simulink library "halout"  (R2021b)
settings: Solver=VariableStepAuto  StartTime=0.0  StopTime=10.0  RelTol=1e-3
undefined symbols (not defined in the file): C_TASK_5MS_S, FALSE, KHAL_CAN1FD1APS3E2E_flg, KHAL_CAN1FD1APS3TxReq_flg, KHAL_CAN1FD1VCU2E2E_flg, KHAL_CAN1FD1VCU2TxReq_flg, KHAL_CAN1FD1VCU3E2E_flg, KHAL_CAN1FD1VCU3TxReq_flg, KHAL_CAN1TxReq_flg, KHAL_CAN1VMCFCM1E2E_flg, KHAL_CAN1VMCFCM1TxReq_flg, KHAL_CAN2TxReq_flg, KHAL_CAN3FD3VCU1toNIDECTxReq_flg, KHAL_CAN3FD3VCU1TxReq_flg, KHAL_CAN3FD3VCU2E2E_flg, KHAL_CAN3FD3VCU2toNIDECE2E_flg, KHAL_CAN3FD3VCU2toNIDECTxReq_flg, KHAL_CAN3FD3VCU2TxReq_flg, KHAL_CAN3TxReq_flg, KHAL_CAN4FD4CE1000E2E_flg, KHAL_CAN4FD4CE1000TxReq_flg, KHAL_CAN4TxReq_flg, KHAL_CAN5TxReq_flg, KHAL_CAN6FD6APS3E2E_flg, KHAL_CAN6FD6APS3TxReq_flg, KHAL_CAN6FD6VCU2E2E_flg, KHAL_CAN6FD6VCU2TxReq_flg, KHAL_CAN6TxReq_flg, ONE_INT, TRUE, ZERO_INT
libraries: FVT_lib x551, simulink x244
(part 12 of 26)

== system halout/HAL_OUT/CAN5/FD5_Debug2_0x4F7 ==
  BSCP_outputs : Inport  OutDataTypeStr=Bus: BSCP_outputs
  BOUTP_outputs : Inport  Port=2  OutDataTypeStr=Bus: BOUTP_outputs
  FDCDKCA0UWBEventSta : Subsystem
  FDCDKCAllowSleepSta : Subsystem
  FDCDKCBLERSSISta : Subsystem
  FDCDKCBLEdcEventSta : Subsystem
  FDCDKCCalDistanceSta : Subsystem
  FDCDKCCommandToBCMCmd : Subsystem
  FDCDKCCoordinateXSta : Subsystem
  FDCDKCCoordinateYSta : Subsystem
  FDCDKCDKeyAreaPESta : Subsystem
  FDCDKCDKeyAreaPSSta : Subsystem
  FDCDKCDKeyAreaPTGSta : Subsystem
  FDCDKCDKeyAreaSPTGSta : Subsystem
  FDCDKCDKeyWelcomeSta : Subsystem
  FDCDKCDkeyAreaRAPSSta : Subsystem
  FDCDKCDkeyShowIVISta : Subsystem
  FDCDKCKeyMissSta : Subsystem
  FDCDKCKeyModeSta : Subsystem
  FDCDKCKeyNumSta : Subsystem
  FDCDKCKeyTypeSta : Subsystem
  FDCDKCOutputPCMDModuleSta : Subsystem
  FDCDKCParkingModeCmd : Subsystem
  FDCDKCReVehDataSta : Subsystem
  FDCDKCRemoLeftPSDCmd : Subsystem
  FDCDKCRemoRightPSDCmd : Subsystem
  FDCDKCSPTGDetCmd : Subsystem
  FDCDKCSPTGOpenCmd : Subsystem
  FDCDKCShippingModeSta : Subsystem
  FDCDKCUIDBatVoltSta : Subsystem
  FDCDKCUIDLowPowerSta : Subsystem
  FDCDKCUWB1DistanceSta : Subsystem
  FDCDKCUWB1FPPSta : Subsystem
  FDCDKCUWB1InvalidSta : Subsystem
  FDCDKCUWB2DistanceSta : Subsystem
  FDCDKCUWB2FPPSta : Subsystem
  FDCDKCUWB2InvalidSta : Subsystem
  FDCDKCUWB3DistanceSta : Subsystem
  FDCDKCUWB3FPPSta : Subsystem
  FDCDKCUWB3InvalidSta : Subsystem
  FDCDKCUWB4DistanceSta : Subsystem
  FDCDKCUWB4FPPSta : Subsystem
  FDCDKCUWB4InvalidSta : Subsystem
  FDCDKCUWB5DistanceSta : Subsystem
  FDCDKCUWB5FPPSta : Subsystem
  FDCDKCUWB5InvalidSta : Subsystem
  FDCDKCUWBDetAreaSta : Subsystem
  FDCDKCUWBDetPTGAreaSta : Subsystem
  FDCDKCUWBOnOffSta : Subsystem
  Ground : Ground
  Ground1 : Ground
  bus_creator : BusCreator  Inputs=47  OutDataTypeStr=Bus: DT_CAN5_SG_FD5_Debug2  NonVirtualBus=on
  bus_selector : BusSelector  OutputSignals=VOUTP_A0UWBEvent_enum
  bus_selector1 : BusSelector  OutputSignals=VOUTP_AllowSleep_flg
  bus_selector10 : BusSelector  OutputSignals=VOUTP_KeyAreaPTG_enum
  bus_selector11 : BusSelector  OutputSignals=VOUTP_KeyAreaSPTGSta_enum
  bus_selector12 : BusSelector  OutputSignals=VOUTP_DKeyWelcomeSta_enum
  bus_selector13 : BusSelector  OutputSignals=VOUTP_DkeyAreaRAPSSta_enum
  bus_selector14 : BusSelector  OutputSignals=VOUTP_DkeyShowIVISta_enum
  bus_selector15 : BusSelector  OutputSignals=VOUTP_KeyMissSta_flg
  bus_selector16 : BusSelector  OutputSignals=VOUTP_KeyModeSta_enum
  bus_selector17 : BusSelector  OutputSignals=VOUTP_KeyNumSta_enum
  bus_selector18 : BusSelector  OutputSignals=VOUTP_KeyTypeSta_enum
  bus_selector19 : BusSelector  OutputSignals=VOUTP_OutputPCMDModule_enum
  bus_selector2 : BusSelector  OutputSignals=VOUTP_BLERSSI_enum
  bus_selector20 : BusSelector  OutputSignals=VOUTP_ParkingModeCmd_enum
  bus_selector21 : BusSelector  OutputSignals=VOUTP_ReVehData_enum
  bus_selector22 : BusSelector  OutputSignals=VOUTP_FDCSPTGDet_flg
  bus_selector23 : BusSelector  OutputSignals=VOUTP_FDCSPTGOpen_flg
  bus_selector24 : BusSelector  OutputSignals=VOUTP_ShippingMode_flg
  bus_selector25 : BusSelector  OutputSignals=VOUTP_UIDBatVolt_enum
  bus_selector26 : BusSelector  OutputSignals=VOUTP_UIDLowPowerSta_flg
  bus_selector27 : BusSelector  OutputSignals=VOUTP_UWB1Distance_enum
  bus_selector28 : BusSelector  OutputSignals=VOUTP_UWB1FPP_enum
  bus_selector29 : BusSelector  OutputSignals=VOUTP_UWB1Invalid_flg
  bus_selector3 : BusSelector  OutputSignals=VOUTP_BLEdcEvent_enum
  bus_selector30 : BusSelector  OutputSignals=VOUTP_UWB2Distance_enum
  bus_selector31 : BusSelector  OutputSignals=VOUTP_UWB2FPP_enum
  bus_selector32 : BusSelector  OutputSignals=VOUTP_UWB2Invalid_flg
  bus_selector33 : BusSelector  OutputSignals=VOUTP_UWB3Distance_enum
  bus_selector34 : BusSelector  OutputSignals=VOUTP_UWB3FPP_enum
  bus_selector35 : BusSelector  OutputSignals=VOUTP_UWB3Invalid_flg
  bus_selector36 : BusSelector  OutputSignals=VOUTP_UWB4Distance_enum
  bus_selector37 : BusSelector  OutputSignals=VOUTP_UWB4FPP_enum
  bus_selector38 : BusSelector  OutputSignals=VOUTP_UWB4Invalid_flg
  bus_selector39 : BusSelector  OutputSignals=VOUTP_UWB0Distance_enum
  bus_selector4 : BusSelector  OutputSignals=VOUTP_CalDistance_enum
  bus_selector40 : BusSelector  OutputSignals=VOUTP_UWB0FPP_enum
  bus_selector41 : BusSelector  OutputSignals=VOUTP_UWB0Invalid_flg
  bus_selector42 : BusSelector  OutputSignals=VOUTP_UWBDetArea_enum
  bus_selector43 : BusSelector  OutputSignals=VOUTP_UWBDetPTGArea_enum
  bus_selector44 : BusSelector  OutputSignals=VOUTP_UWBOnOff_flg
  bus_selector5 : BusSelector  OutputSignals=VOUTP_PCommandToBCM_enum
  bus_selector6 : BusSelector  OutputSignals=VOUTP_CoordinateX_enum
  bus_selector7 : BusSelector  OutputSignals=VOUTP_CoordinateY_enum
  bus_selector8 : BusSelector  OutputSignals=VOUTP_KeyAreaLockUnlock_enum
  bus_selector9 : BusSelector  OutputSignals=VOUTP_KeyAreaPS_enum
  FD5_Debug2 : Outport
  wires:
  BSCP_outputs/1 -> [BSCP_outputs]
  BOUTP_outputs/1 -> [BOUTP_outputs]
  [CAN5_FDC_DKC_A0_UWB_Event_Sta] -> bus_creator/1  "CAN5_FDC_DKC_A0_UWB_Event_Sta"
  [CAN5_FDC_DKC_AllowSleep_Sta] -> bus_creator/2  "CAN5_FDC_DKC_AllowSleep_Sta"
  [CAN5_FDC_DKC_BLERSSI_Sta] -> bus_creator/3  "CAN5_FDC_DKC_BLERSSI_Sta"
  [CAN5_FDC_DKC_BLEdcEvent_Sta] -> bus_creator/4  "CAN5_FDC_DKC_BLEdcEvent_Sta"
  [CAN5_FDC_DKC_CalDistance_Sta] -> bus_creator/5  "CAN5_FDC_DKC_CalDistance_Sta"
  [CAN5_FDC_DKC_CommandToBCM_Cmd] -> bus_creator/6  "CAN5_FDC_DKC_CommandToBCM_Cmd"
  [CAN5_FDC_DKC_CoordinateX_Sta] -> bus_creator/7  "CAN5_FDC_DKC_CoordinateX_Sta"
  [CAN5_FDC_DKC_CoordinateY_Sta] -> bus_creator/8  "CAN5_FDC_DKC_CoordinateY_Sta"
  [CAN5_FDC_DKC_DKeyAreaPE_Sta] -> bus_creator/9  "CAN5_FDC_DKC_DKeyAreaPE_Sta"
  [CAN5_FDC_DKC_DKeyAreaPS_Sta] -> bus_creator/10  "CAN5_FDC_DKC_DKeyAreaPS_Sta"
  [CAN5_FDC_DKC_DKeyAreaPTG_Sta] -> bus_creator/11  "CAN5_FDC_DKC_DKeyAreaPTG_Sta"
  [CAN5_FDC_DKC_DKeyAreaSPTG_Sta] -> bus_creator/12  "CAN5_FDC_DKC_DKeyAreaSPTG_Sta"
  [CAN5_FDC_DKC_DKeyWelcome_Sta] -> bus_creator/13  "CAN5_FDC_DKC_DKeyWelcome_Sta"
  [CAN5_FDC_DKC_DkeyAreaRAPS_Sta] -> bus_creator/14  "CAN5_FDC_DKC_DkeyAreaRAPS_Sta"
  [CAN5_FDC_DKC_DkeyShowIVI_Sta] -> bus_creator/15  "CAN5_FDC_DKC_DkeyShowIVI_Sta"
  [CAN5_FDC_DKC_KeyMiss_Sta] -> bus_creator/16  "CAN5_FDC_DKC_KeyMiss_Sta"
  [CAN5_FDC_DKC_KeyMode_Sta] -> bus_creator/17  "CAN5_FDC_DKC_KeyMode_Sta"
  [CAN5_FDC_DKC_KeyNum_Sta] -> bus_creator/18  "CAN5_FDC_DKC_KeyNum_Sta"
  [CAN5_FDC_DKC_KeyType_Sta] -> bus_creator/19  "CAN5_FDC_DKC_KeyType_Sta"
  [CAN5_FDC_DKC_OutputPCMDModule_Sta] -> bus_creator/20  "CAN5_FDC_DKC_OutputPCMDModule_Sta"
  [CAN5_FDC_DKC_ParkingMode_Cmd] -> bus_creator/21  "CAN5_FDC_DKC_ParkingMode_Cmd"
  [CAN5_FDC_DKC_ReVehData_Sta] -> bus_creator/22  "CAN5_FDC_DKC_ReVehData_Sta"
  [CAN5_FDC_DKC_RemoLeftPSD_Cmd] -> bus_creator/23  "CAN5_FDC_DKC_RemoLeftPSD_Cmd"
  [CAN5_FDC_DKC_RemoRightPSD_Cmd] -> bus_creator/24  "CAN5_FDC_DKC_RemoRightPSD_Cmd"
  [CAN5_FDC_DKC_SPTGDet_Cmd] -> bus_creator/25  "CAN5_FDC_DKC_SPTGDet_Cmd"
  [CAN5_FDC_DKC_SPTGOpen_Cmd] -> bus_creator/26  "CAN5_FDC_DKC_SPTGOpen_Cmd"
  [CAN5_FDC_DKC_ShippingMode_Sta] -> bus_creator/27  "CAN5_FDC_DKC_ShippingMode_Sta"
  [CAN5_FDC_DKC_UIDBatVolt_Sta] -> bus_creator/28  "CAN5_FDC_DKC_UIDBatVolt_Sta"
  [CAN5_FDC_DKC_UIDLowPower_Sta] -> bus_creator/29  "CAN5_FDC_DKC_UIDLowPower_Sta"
  [CAN5_FDC_DKC_UWB1_Distance_Sta] -> bus_creator/30  "CAN5_FDC_DKC_UWB1_Distance_Sta"
  [CAN5_FDC_DKC_UWB1_FPP_Sta] -> bus_creator/31  "CAN5_FDC_DKC_UWB1_FPP_Sta"
  [CAN5_FDC_DKC_UWB1_Invalid_Sta] -> bus_creator/32  "CAN5_FDC_DKC_UWB1_Invalid_Sta"
  [CAN5_FDC_DKC_UWB2_Distance_Sta] -> bus_creator/33  "CAN5_FDC_DKC_UWB2_Distance_Sta"
  [CAN5_FDC_DKC_UWB2_FPP_Sta] -> bus_creator/34  "CAN5_FDC_DKC_UWB2_FPP_Sta"
  [CAN5_FDC_DKC_UWB2_Invalid_Sta] -> bus_creator/35  "CAN5_FDC_DKC_UWB2_Invalid_Sta"
  [CAN5_FDC_DKC_UWB3_Distance_Sta] -> bus_creator/36  "CAN5_FDC_DKC_UWB3_Distance_Sta"
  [CAN5_FDC_DKC_UWB3_FPP_Sta] -> bus_creator/37  "CAN5_FDC_DKC_UWB3_FPP_Sta"
  [CAN5_FDC_DKC_UWB3_Invalid_Sta] -> bus_creator/38  "CAN5_FDC_DKC_UWB3_Invalid_Sta"
  [CAN5_FDC_DKC_UWB4_Distance_Sta] -> bus_creator/39  "CAN5_FDC_DKC_UWB4_Distance_Sta"
  [CAN5_FDC_DKC_UWB4_FPP_Sta] -> bus_creator/40  "CAN5_FDC_DKC_UWB4_FPP_Sta"
  [CAN5_FDC_DKC_UWB4_Invalid_Sta] -> bus_creator/41  "CAN5_FDC_DKC_UWB4_Invalid_Sta"
  [CAN5_FDC_DKC_UWB5_Distance_Sta] -> bus_creator/42  "CAN5_FDC_DKC_UWB5_Distance_Sta"
  [CAN5_FDC_DKC_UWB5_FPP_Sta] -> bus_creator/43  "CAN5_FDC_DKC_UWB5_FPP_Sta"
  [CAN5_FDC_DKC_UWB5_Invalid_Sta] -> bus_creator/44  "CAN5_FDC_DKC_UWB5_Invalid_Sta"
  [CAN5_FDC_DKC_UWBDetArea_Sta] -> bus_creator/45  "CAN5_FDC_DKC_UWBDetArea_Sta"
  [CAN5_FDC_DKC_UWBDetPTGArea_Sta] -> bus_creator/46  "CAN5_FDC_DKC_UWBDetPTGArea_Sta"
  [CAN5_FDC_DKC_UWB_OnOff_Sta] -> bus_creator/47  "CAN5_FDC_DKC_UWB_OnOff_Sta"
  bus_creator/1 -> FD5_Debug2/1
  FDCDKCA0UWBEventSta/1(CAN5_FDC_DKC_A0_UWB_Event_Sta) -> [CAN5_FDC_DKC_A0_UWB_Event_Sta]
  FDCDKCAllowSleepSta/1(CAN5_FDC_DKC_AllowSleep_Sta) -> [CAN5_FDC_DKC_AllowSleep_Sta]
  FDCDKCBLERSSISta/1(CAN5_FDC_DKC_BLERSSI_Sta) -> [CAN5_FDC_DKC_BLERSSI_Sta]
  FDCDKCBLEdcEventSta/1(CAN5_FDC_DKC_BLEdcEvent_Sta) -> [CAN5_FDC_DKC_BLEdcEvent_Sta]
  FDCDKCCalDistanceSta/1(CAN5_FDC_DKC_CalDistance_Sta) -> [CAN5_FDC_DKC_CalDistance_Sta]
  FDCDKCCommandToBCMCmd/1(CAN5_FDC_DKC_CommandToBCM_Cmd) -> [CAN5_FDC_DKC_CommandToBCM_Cmd]
  FDCDKCCoordinateXSta/1(CAN5_FDC_DKC_CoordinateX_Sta) -> [CAN5_FDC_DKC_CoordinateX_Sta]
  FDCDKCCoordinateYSta/1(CAN5_FDC_DKC_CoordinateY_Sta) -> [CAN5_FDC_DKC_CoordinateY_Sta]
  FDCDKCDKeyAreaPESta/1(CAN5_FDC_DKC_DKeyAreaPE_Sta) -> [CAN5_FDC_DKC_DKeyAreaPE_Sta]
  FDCDKCDKeyAreaPSSta/1(CAN5_FDC_DKC_DKeyAreaPS_Sta) -> [CAN5_FDC_DKC_DKeyAreaPS_Sta]
  FDCDKCDKeyAreaPTGSta/1(CAN5_FDC_DKC_DKeyAreaPTG_Sta) -> [CAN5_FDC_DKC_DKeyAreaPTG_Sta]
  FDCDKCDKeyAreaSPTGSta/1(CAN5_FDC_DKC_DKeyAreaSPTG_Sta) -> [CAN5_FDC_DKC_DKeyAreaSPTG_Sta]
  FDCDKCDKeyWelcomeSta/1(CAN5_FDC_DKC_DKeyWelcome_Sta) -> [CAN5_FDC_DKC_DKeyWelcome_Sta]
  FDCDKCDkeyAreaRAPSSta/1(CAN5_FDC_DKC_DkeyAreaRAPS_Sta) -> [CAN5_FDC_DKC_DkeyAreaRAPS_Sta]
  FDCDKCDkeyShowIVISta/1(CAN5_FDC_DKC_DkeyShowIVI_Sta) -> [CAN5_FDC_DKC_DkeyShowIVI_Sta]
  FDCDKCKeyMissSta/1(CAN5_FDC_DKC_KeyMiss_Sta) -> [CAN5_FDC_DKC_KeyMiss_Sta]
  FDCDKCKeyModeSta/1(CAN5_FDC_DKC_KeyMode_Sta) -> [CAN5_FDC_DKC_KeyMode_Sta]
  FDCDKCKeyNumSta/1(CAN5_FDC_DKC_KeyNum_Sta) -> [CAN5_FDC_DKC_KeyNum_Sta]
  FDCDKCKeyTypeSta/1(CAN5_FDC_DKC_KeyType_Sta) -> [CAN5_FDC_DKC_KeyType_Sta]
  FDCDKCOutputPCMDModuleSta/1(CAN5_FDC_DKC_OutputPCMDModule_Sta) -> [CAN5_FDC_DKC_OutputPCMDModule_Sta]
  FDCDKCParkingModeCmd/1(CAN5_FDC_DKC_ParkingMode_Cmd) -> [CAN5_FDC_DKC_ParkingMode_Cmd]
  FDCDKCReVehDataSta/1(CAN5_FDC_DKC_ReVehData_Sta) -> [CAN5_FDC_DKC_ReVehData_Sta]
  FDCDKCRemoLeftPSDCmd/1(CAN5_FDC_DKC_RemoLeftPSD_Cmd) -> [CAN5_FDC_DKC_RemoLeftPSD_Cmd]
  FDCDKCRemoRightPSDCmd/1(CAN5_FDC_DKC_RemoRightPSD_Cmd) -> [CAN5_FDC_DKC_RemoRightPSD_Cmd]
  FDCDKCSPTGDetCmd/1(CAN5_FDC_DKC_SPTGDet_Cmd) -> [CAN5_FDC_DKC_SPTGDet_Cmd]
  FDCDKCSPTGOpenCmd/1(CAN5_FDC_DKC_SPTGOpen_Cmd) -> [CAN5_FDC_DKC_SPTGOpen_Cmd]
  FDCDKCShippingModeSta/1(CAN5_FDC_DKC_ShippingMode_Sta) -> [CAN5_FDC_DKC_ShippingMode_Sta]
  FDCDKCUIDBatVoltSta/1(CAN5_FDC_DKC_UIDBatVolt_Sta) -> [CAN5_FDC_DKC_UIDBatVolt_Sta]
  FDCDKCUIDLowPowerSta/1(CAN5_FDC_DKC_UIDLowPower_Sta) -> [CAN5_FDC_DKC_UIDLowPower_Sta]
  FDCDKCUWB1DistanceSta/1(CAN5_FDC_DKC_UWB1_Distance_Sta) -> [CAN5_FDC_DKC_UWB1_Distance_Sta]
  FDCDKCUWB1FPPSta/1(CAN5_FDC_DKC_UWB1_FPP_Sta) -> [CAN5_FDC_DKC_UWB1_FPP_Sta]
  FDCDKCUWB1InvalidSta/1(CAN5_FDC_DKC_UWB1_Invalid_Sta) -> [CAN5_FDC_DKC_UWB1_Invalid_Sta]
  FDCDKCUWB2DistanceSta/1(CAN5_FDC_DKC_UWB2_Distance_Sta) -> [CAN5_FDC_DKC_UWB2_Distance_Sta]
  FDCDKCUWB2FPPSta/1(CAN5_FDC_DKC_UWB2_FPP_Sta) -> [CAN5_FDC_DKC_UWB2_FPP_Sta]
  FDCDKCUWB2InvalidSta/1(CAN5_FDC_DKC_UWB2_Invalid_Sta) -> [CAN5_FDC_DKC_UWB2_Invalid_Sta]
  FDCDKCUWB3DistanceSta/1(CAN5_FDC_DKC_UWB3_Distance_Sta) -> [CAN5_FDC_DKC_UWB3_Distance_Sta]
  FDCDKCUWB3FPPSta/1(CAN5_FDC_DKC_UWB3_FPP_Sta) -> [CAN5_FDC_DKC_UWB3_FPP_Sta]
  FDCDKCUWB3InvalidSta/1(CAN5_FDC_DKC_UWB3_Invalid_Sta) -> [CAN5_FDC_DKC_UWB3_Invalid_Sta]
  FDCDKCUWB4DistanceSta/1(CAN5_FDC_DKC_UWB4_Distance_Sta) -> [CAN5_FDC_DKC_UWB4_Distance_Sta]
  FDCDKCUWB4FPPSta/1(CAN5_FDC_DKC_UWB4_FPP_Sta) -> [CAN5_FDC_DKC_UWB4_FPP_Sta]
  FDCDKCUWB4InvalidSta/1(CAN5_FDC_DKC_UWB4_Invalid_Sta) -> [CAN5_FDC_DKC_UWB4_Invalid_Sta]
  FDCDKCUWB5DistanceSta/1(CAN5_FDC_DKC_UWB5_Distance_Sta) -> [CAN5_FDC_DKC_UWB5_Distance_Sta]
  FDCDKCUWB5FPPSta/1(CAN5_FDC_DKC_UWB5_FPP_Sta) -> [CAN5_FDC_DKC_UWB5_FPP_Sta]
  FDCDKCUWB5InvalidSta/1(CAN5_FDC_DKC_UWB5_Invalid_Sta) -> [CAN5_FDC_DKC_UWB5_Invalid_Sta]
  FDCDKCUWBDetAreaSta/1(CAN5_FDC_DKC_UWBDetArea_Sta) -> [CAN5_FDC_DKC_UWBDetArea_Sta]
  FDCDKCUWBDetPTGAreaSta/1(CAN5_FDC_DKC_UWBDetPTGArea_Sta) -> [CAN5_FDC_DKC_UWBDetPTGArea_Sta]
  FDCDKCUWBOnOffSta/1(CAN5_FDC_DKC_UWB_OnOff_Sta) -> [CAN5_FDC_DKC_UWB_OnOff_Sta]
  bus_selector/1 -> FDCDKCA0UWBEventSta/1(FDCDKCA0UWBEventSta)  "<VOUTP_A0UWBEvent_enum>"
  [BOUTP_outputs] -> bus_selector/1
  bus_selector1/1 -> FDCDKCAllowSleepSta/1(FDCDKCAllowSleepSta)  "<VOUTP_AllowSleep_flg>"
  [BOUTP_outputs] -> bus_selector1/1
  bus_selector2/1 -> FDCDKCBLERSSISta/1(FDCDKCBLERSSISta)  "<VOUTP_BLERSSI_enum>"
  [BOUTP_outputs] -> bus_selector2/1
  bus_selector3/1 -> FDCDKCBLEdcEventSta/1(FDCDKCBLEdcEventSta)  "<VOUTP_BLEdcEvent_enum>"
  [BOUTP_outputs] -> bus_selector3/1
  bus_selector4/1 -> FDCDKCCalDistanceSta/1(FDCDKCCalDistanceSta)  "<VOUTP_CalDistance_enum>"
  [BOUTP_outputs] -> bus_selector4/1
  bus_selector5/1 -> FDCDKCCommandToBCMCmd/1(FDCDKCCommandToBCMCmd)  "<VOUTP_PCommandToBCM_enum>"
  [BOUTP_outputs] -> bus_selector5/1
  bus_selector6/1 -> FDCDKCCoordinateXSta/1(FDCDKCCoordinateXSta)  "<VOUTP_CoordinateX_enum>"
  [BOUTP_outputs] -> bus_selector6/1
  bus_selector7/1 -> FDCDKCCoordinateYSta/1(FDCDKCCoordinateYSta)  "<VOUTP_CoordinateY_enum>"
  [BOUTP_outputs] -> bus_selector7/1
  bus_selector8/1 -> FDCDKCDKeyAreaPESta/1(FDCDKCDKeyAreaPESta)  "<VOUTP_KeyAreaLockUnlock_enum>"
  [BOUTP_outputs] -> bus_selector8/1
  bus_selector9/1 -> FDCDKCDKeyAreaPSSta/1(FDCDKCDKeyAreaPSSta)  "<VOUTP_KeyAreaPS_enum>"
  [BOUTP_outputs] -> bus_selector9/1
  bus_selector10/1 -> FDCDKCDKeyAreaPTGSta/1(FDCDKCDKeyAreaPTGSta)  "<VOUTP_KeyAreaPTG_enum>"
  [BOUTP_outputs] -> bus_selector10/1
  bus_selector11/1 -> FDCDKCDKeyAreaSPTGSta/1(FDCDKCDKeyAreaSPTGSta)  "<VOUTP_KeyAreaSPTGSta_enum>"
  [BOUTP_outputs] -> bus_selector11/1
  bus_selector12/1 -> FDCDKCDKeyWelcomeSta/1(FDCDKCDKeyWelcomeSta)  "<VOUTP_DKeyWelcomeSta_enum>"
  [BOUTP_outputs] -> bus_selector12/1
  bus_selector13/1 -> FDCDKCDkeyAreaRAPSSta/1(FDCDKCDkeyAreaRAPSSta)  "<VOUTP_DkeyAreaRAPSSta_enum>"
  [BOUTP_outputs] -> bus_selector13/1
  bus_selector14/1 -> FDCDKCDkeyShowIVISta/1(FDCDKCDkeyShowIVISta)  "<VOUTP_DkeyShowIVISta_enum>"
  [BOUTP_outputs] -> bus_selector14/1
  bus_selector15/1 -> FDCDKCKeyMissSta/1(FDCDKCKeyMissSta)  "<VOUTP_KeyMissSta_flg>"
  [BOUTP_outputs] -> bus_selector15/1
  bus_selector16/1 -> FDCDKCKeyModeSta/1(FDCDKCKeyModeSta)  "<VOUTP_KeyModeSta_enum>"
  [BOUTP_outputs] -> bus_selector16/1
  bus_selector17/1 -> FDCDKCKeyNumSta/1(FDCDKCKeyNumSta)  "<VOUTP_KeyNumSta_enum>"
  [BOUTP_outputs] -> bus_selector17/1
  bus_selector18/1 -> FDCDKCKeyTypeSta/1(FDCDKCKeyTypeSta)  "<VOUTP_KeyTypeSta_enum>"
  [BOUTP_outputs] -> bus_selector18/1
  bus_selector19/1 -> FDCDKCOutputPCMDModuleSta/1(FDCDKCOutputPCMDModuleSta)  "<VOUTP_OutputPCMDModule_enum>"
  [BOUTP_outputs] -> bus_selector19/1
  bus_selector20/1 -> FDCDKCParkingModeCmd/1(FDCDKCParkingModeCmd)  "<VOUTP_ParkingModeCmd_enum>"
  [BOUTP_outputs] -> bus_selector20/1
  bus_selector21/1 -> FDCDKCReVehDataSta/1(FDCDKCReVehDataSta)  "<VOUTP_ReVehData_enum>"
  [BOUTP_outputs] -> bus_selector21/1
  Ground/1 -> FDCDKCRemoLeftPSDCmd/1(FDCDKCRemoLeftPSDCmd)
  Ground1/1 -> FDCDKCRemoRightPSDCmd/1(FDCDKCRemoRightPSDCmd)
  bus_selector22/1 -> FDCDKCSPTGDetCmd/1(FDCDKCSPTGDetCmd)  "<VOUTP_FDCSPTGDet_flg>"
  [BOUTP_outputs] -> bus_selector22/1
  bus_selector23/1 -> FDCDKCSPTGOpenCmd/1(FDCDKCSPTGOpenCmd)  "<VOUTP_FDCSPTGOpen_flg>"
  [BOUTP_outputs] -> bus_selector23/1
  bus_selector24/1 -> FDCDKCShippingModeSta/1(FDCDKCShippingModeSta)  "<VOUTP_ShippingMode_flg>"
  [BOUTP_outputs] -> bus_selector24/1
  bus_selector25/1 -> FDCDKCUIDBatVoltSta/1(FDCDKCUIDBatVoltSta)  "<VOUTP_UIDBatVolt_enum>"
  [BOUTP_outputs] -> bus_selector25/1
  bus_selector26/1 -> FDCDKCUIDLowPowerSta/1(FDCDKCUIDLowPowerSta)  "<VOUTP_UIDLowPowerSta_flg>"
  [BOUTP_outputs] -> bus_selector26/1
  bus_selector27/1 -> FDCDKCUWB1DistanceSta/1(FDCDKCUWB1DistanceSta)  "<VOUTP_UWB1Distance_enum>"
  [BOUTP_outputs] -> bus_selector27/1
  bus_selector28/1 -> FDCDKCUWB1FPPSta/1(FDCDKCUWB1FPPSta)  "<VOUTP_UWB1FPP_enum>"
  [BOUTP_outputs] -> bus_selector28/1
  bus_selector29/1 -> FDCDKCUWB1InvalidSta/1(FDCDKCUWB1InvalidSta)  "<VOUTP_UWB1Invalid_flg>"
  [BOUTP_outputs] -> bus_selector29/1
  bus_selector30/1 -> FDCDKCUWB2DistanceSta/1(FDCDKCUWB2DistanceSta)  "<VOUTP_UWB2Distance_enum>"
  [BOUTP_outputs] -> bus_selector30/1
  bus_selector31/1 -> FDCDKCUWB2FPPSta/1(FDCDKCUWB2FPPSta)  "<VOUTP_UWB2FPP_enum>"
  [BOUTP_outputs] -> bus_selector31/1
  bus_selector32/1 -> FDCDKCUWB2InvalidSta/1(FDCDKCUWB2InvalidSta)  "<VOUTP_UWB2Invalid_flg>"
  [BOUTP_outputs] -> bus_selector32/1
  bus_selector33/1 -> FDCDKCUWB3DistanceSta/1(FDCDKCUWB3DistanceSta)  "<VOUTP_UWB3Distance_enum>"
  [BOUTP_outputs] -> bus_selector33/1
  bus_selector34/1 -> FDCDKCUWB3FPPSta/1(FDCDKCUWB3FPPSta)  "<VOUTP_UWB3FPP_enum>"
  [BOUTP_outputs] -> bus_selector34/1
  bus_selector35/1 -> FDCDKCUWB3InvalidSta/1(FDCDKCUWB3InvalidSta)  "<VOUTP_UWB3Invalid_flg>"
  [BOUTP_outputs] -> bus_selector35/1
  bus_selector36/1 -> FDCDKCUWB4DistanceSta/1(FDCDKCUWB4DistanceSta)  "<VOUTP_UWB4Distance_enum>"
  [BOUTP_outputs] -> bus_selector36/1
  bus_selector37/1 -> FDCDKCUWB4FPPSta/1(FDCDKCUWB4FPPSta)  "<VOUTP_UWB4FPP_enum>"
  [BOUTP_outputs] -> bus_selector37/1
  bus_selector38/1 -> FDCDKCUWB4InvalidSta/1(FDCDKCUWB4InvalidSta)  "<VOUTP_UWB4Invalid_flg>"
  [BOUTP_outputs] -> bus_selector38/1
  bus_selector39/1 -> FDCDKCUWB5DistanceSta/1(FDCDKCUWB5DistanceSta)  "<VOUTP_UWB0Distance_enum>"
  [BOUTP_outputs] -> bus_selector39/1
  bus_selector40/1 -> FDCDKCUWB5FPPSta/1(FDCDKCUWB5FPPSta)  "<VOUTP_UWB0FPP_enum>"
  [BOUTP_outputs] -> bus_selector40/1
  bus_selector41/1 -> FDCDKCUWB5InvalidSta/1(FDCDKCUWB5InvalidSta)  "<VOUTP_UWB0Invalid_flg>"
  [BOUTP_outputs] -> bus_selector41/1
  bus_selector42/1 -> FDCDKCUWBDetAreaSta/1(FDCDKCUWBDetAreaSta)  "<VOUTP_UWBDetArea_enum>"
  [BOUTP_outputs] -> bus_selector42/1
  bus_selector43/1 -> FDCDKCUWBDetPTGAreaSta/1(FDCDKCUWBDetPTGAreaSta)  "<VOUTP_UWBDetPTGArea_enum>"
  [BOUTP_outputs] -> bus_selector43/1
  bus_selector44/1 -> FDCDKCUWBOnOffSta/1(FDCDKCUWBOnOffSta)  "<VOUTP_UWBOnOff_flg>"
  [BOUTP_outputs] -> bus_selector44/1

== system halout/HAL_OUT/CAN5/FD5_Debug3_0x4F3 ==
  BSCP_outputs : Inport  OutDataTypeStr=Bus: BSCP_outputs
  BOUTP_outputs : Inport  Port=2  OutDataTypeStr=Bus: BOUTP_outputs
  FDCVMCActReqAccCmd : Subsystem
  FDCVMCExtraMSACtrlSta : Subsystem
  FDCVMCIMUGxCmd : Subsystem
  FDCVMCIMUGyCmd : Subsystem
  FDCVMCIMUGzCmd : Subsystem
  FDCVMCIMUPitchRateCmd : Subsystem
  FDCVMCIMURollRateCmd : Subsystem
  FDCVMCIMUYawRateCmd : Subsystem
  FDCVMCLongAccelCmd : Subsystem
  bus_creator : BusCreator  Inputs=9  OutDataTypeStr=Bus: DT_CAN5_SG_FD5_Debug3  NonVirtualBus=on
  bus_selector : BusSelector  OutputSignals=VOUTP_ActACCRequiredAccel_mps2
  bus_selector1 : BusSelector  OutputSignals=VOUTP_ExtraMSACtrlSta_enum
  bus_selector2 : BusSelector  OutputSignals=VOUTP_CalibratedAccX_G
  bus_selector3 : BusSelector  OutputSignals=VOUTP_CalibratedAccY_G
  bus_selector4 : BusSelector  OutputSignals=VOUTP_CalibratedAccZ_G
  bus_selector5 : BusSelector  OutputSignals=VOUTP_CalibratedGyroY_Dps
  bus_selector6 : BusSelector  OutputSignals=VOUTP_CalibratedGyroX_Dps
  bus_selector7 : BusSelector  OutputSignals=VOUTP_CalibratedGyroZ_Dps
  bus_selector8 : BusSelector  OutputSignals=VOUTP_LongAcc_Gps
  FD5_Debug3 : Outport
  wires:
  BSCP_outputs/1 -> [BSCP_outputs]
  BOUTP_outputs/1 -> [BOUTP_outputs]
  [CAN5_FDC_VMC_ActReqAcc_Cmd] -> bus_creator/1  "CAN5_FDC_VMC_ActReqAcc_Cmd"
  [CAN5_FDC_VMC_ExtraMSACtrl_Sta] -> bus_creator/2  "CAN5_FDC_VMC_ExtraMSACtrl_Sta"
  [CAN5_FDC_VMC_IMUGx_Cmd] -> bus_creator/3  "CAN5_FDC_VMC_IMUGx_Cmd"
  [CAN5_FDC_VMC_IMUGy_Cmd] -> bus_creator/4  "CAN5_FDC_VMC_IMUGy_Cmd"
  [CAN5_FDC_VMC_IMUGz_Cmd] -> bus_creator/5  "CAN5_FDC_VMC_IMUGz_Cmd"
  [CAN5_FDC_VMC_IMUPitchRate_Cmd] -> bus_creator/6  "CAN5_FDC_VMC_IMUPitchRate_Cmd"
  [CAN5_FDC_VMC_IMURollRate_Cmd] -> bus_creator/7  "CAN5_FDC_VMC_IMURollRate_Cmd"
  [CAN5_FDC_VMC_IMUYawRate_Cmd] -> bus_creator/8  "CAN5_FDC_VMC_IMUYawRate_Cmd"
  [CAN5_FDC_VMC_LongAccel_Cmd] -> bus_creator/9  "CAN5_FDC_VMC_LongAccel_Cmd"
  bus_creator/1 -> FD5_Debug3/1
  FDCVMCActReqAccCmd/1(CAN5_FDC_VMC_ActReqAcc_Cmd) -> [CAN5_FDC_VMC_ActReqAcc_Cmd]
  FDCVMCExtraMSACtrlSta/1(CAN5_FDC_VMC_ExtraMSACtrl_Sta) -> [CAN5_FDC_VMC_ExtraMSACtrl_Sta]
  FDCVMCIMUGxCmd/1(CAN5_FDC_VMC_IMUGx_Cmd) -> [CAN5_FDC_VMC_IMUGx_Cmd]
  FDCVMCIMUGyCmd/1(CAN5_FDC_VMC_IMUGy_Cmd) -> [CAN5_FDC_VMC_IMUGy_Cmd]
  FDCVMCIMUGzCmd/1(CAN5_FDC_VMC_IMUGz_Cmd) -> [CAN5_FDC_VMC_IMUGz_Cmd]
  FDCVMCIMUPitchRateCmd/1(CAN5_FDC_VMC_IMUPitchRate_Cmd) -> [CAN5_FDC_VMC_IMUPitchRate_Cmd]
  FDCVMCIMURollRateCmd/1(CAN5_FDC_VMC_IMURollRate_Cmd) -> [CAN5_FDC_VMC_IMURollRate_Cmd]
  FDCVMCIMUYawRateCmd/1(CAN5_FDC_VMC_IMUYawRate_Cmd) -> [CAN5_FDC_VMC_IMUYawRate_Cmd]
  FDCVMCLongAccelCmd/1(CAN5_FDC_VMC_LongAccel_Cmd) -> [CAN5_FDC_VMC_LongAccel_Cmd]
  bus_selector/1 -> FDCVMCActReqAccCmd/1(FDCVMCActReqAccCmd)  "<VOUTP_ActACCRequiredAccel_mps2>"
  [BOUTP_outputs] -> bus_selector/1
  bus_selector1/1 -> FDCVMCExtraMSACtrlSta/1(FDCVMCExtraMSACtrlSta)  "<VOUTP_ExtraMSACtrlSta_enum>"
  [BOUTP_outputs] -> bus_selector1/1
  bus_selector2/1 -> FDCVMCIMUGxCmd/1(FDCVMCIMUGxCmd)  "<VOUTP_CalibratedAccX_G>"
  [BOUTP_outputs] -> bus_selector2/1
  bus_selector3/1 -> FDCVMCIMUGyCmd/1(FDCVMCIMUGyCmd)  "<VOUTP_CalibratedAccY_G>"
  [BOUTP_outputs] -> bus_selector3/1
  bus_selector4/1 -> FDCVMCIMUGzCmd/1(FDCVMCIMUGzCmd)  "<VOUTP_CalibratedAccZ_G>"
  [BOUTP_outputs] -> bus_selector4/1
  bus_selector5/1 -> FDCVMCIMUPitchRateCmd/1(FDCVMCIMUPitchRateCmd)  "<VOUTP_CalibratedGyroY_Dps>"
  [BOUTP_outputs] -> bus_selector5/1
  bus_selector6/1 -> FDCVMCIMURollRateCmd/1(FDCVMCIMURollRateCmd)  "<VOUTP_CalibratedGyroX_Dps>"
  [BOUTP_outputs] -> bus_selector6/1
  bus_selector7/1 -> FDCVMCIMUYawRateCmd/1(FDCVMCIMUYawRateCmd)  "<VOUTP_CalibratedGyroZ_Dps>"
  [BOUTP_outputs] -> bus_selector7/1
  bus_selector8/1 -> FDCVMCLongAccelCmd/1(FDCVMCLongAccelCmd)  "<VOUTP_LongAcc_Gps>"
  [BOUTP_outputs] -> bus_selector8/1

== system halout/HAL_OUT/CAN5/GW5_CE100_0_0x1C5 ==
  BSCP_outputs : Inport  OutDataTypeStr=Bus: BSCP_outputs
  BOUTP_outputs : Inport  Port=2  OutDataTypeStr=Bus: BOUTP_outputs
  FDCBCMWinLFOpenedSta : Subsystem
  FDCBCMWinLROpenedSta : Subsystem
  FDCBCMWinRFOpenedSta : Subsystem
  FDCBCMWinRROpenedSta : Subsystem
  bus_creator : BusCreator  Inputs=4  OutDataTypeStr=Bus: DT_CAN5_SG_GW5_CE100_0  NonVirtualBus=on
  bus_selector : BusSelector  OutputSignals=VOUTP_WinLFOpenedSta_pct
  bus_selector1 : BusSelector  OutputSignals=VOUTP_WinLROpenedSta_pct
  bus_selector2 : BusSelector  OutputSignals=VOUTP_WinRFOpenedSta_pct
  bus_selector3 : BusSelector  OutputSignals=VOUTP_WinRROpenedSta_pct
  GW5_CE100_0 : Outport
  wires:
  BSCP_outputs/1 -> [BSCP_outputs]
  BOUTP_outputs/1 -> [BOUTP_outputs]
  [CAN5_FDC_BCM_WinLFOpened_Sta] -> bus_creator/1  "CAN5_FDC_BCM_WinLFOpened_Sta"
  [CAN5_FDC_BCM_WinLROpened_Sta] -> bus_creator/2  "CAN5_FDC_BCM_WinLROpened_Sta"
  [CAN5_FDC_BCM_WinRFOpened_Sta] -> bus_creator/3  "CAN5_FDC_BCM_WinRFOpened_Sta"
  [CAN5_FDC_BCM_WinRROpened_Sta] -> bus_creator/4  "CAN5_FDC_BCM_WinRROpened_Sta"
  bus_creator/1 -> GW5_CE100_0/1
  FDCBCMWinLFOpenedSta/1(CAN5_FDC_BCM_WinLFOpened_Sta) -> [CAN5_FDC_BCM_WinLFOpened_Sta]
  FDCBCMWinLROpenedSta/1(CAN5_FDC_BCM_WinLROpened_Sta) -> [CAN5_FDC_BCM_WinLROpened_Sta]
  FDCBCMWinRFOpenedSta/1(CAN5_FDC_BCM_WinRFOpened_Sta) -> [CAN5_FDC_BCM_WinRFOpened_Sta]
  FDCBCMWinRROpenedSta/1(CAN5_FDC_BCM_WinRROpened_Sta) -> [CAN5_FDC_BCM_WinRROpened_Sta]
  bus_selector/1 -> FDCBCMWinLFOpenedSta/1(FDCBCMWinLFOpenedSta)  "<VOUTP_WinLFOpenedSta_pct>"
  [BOUTP_outputs] -> bus_selector/1
  bus_selector1/1 -> FDCBCMWinLROpenedSta/1(FDCBCMWinLROpenedSta)  "<VOUTP_WinLROpenedSta_pct>"
  [BOUTP_outputs] -> bus_selector1/1
  bus_selector2/1 -> FDCBCMWinRFOpenedSta/1(FDCBCMWinRFOpenedSta)  "<VOUTP_WinRFOpenedSta_pct>"
  [BOUTP_outputs] -> bus_selector2/1
  bus_selector3/1 -> FDCBCMWinRROpenedSta/1(FDCBCMWinRROpenedSta)  "<VOUTP_WinRROpenedSta_pct>"
  [BOUTP_outputs] -> bus_selector3/1

== system halout/HAL_OUT/CAN6/FD6_APS3_0x238 ==
  BSCP_outputs : Inport  OutDataTypeStr=Bus: BSCP_outputs
  BOUTP_outputs : Inport  Port=2  OutDataTypeStr=Bus: BOUTP_outputs
  Trigger : TriggerPort  TriggerType=function-call  VariantControl=(inherit)
  APS3LifeCount : Subsystem
  APS3checksum : Subsystem
  APSDecReq : Subsystem
  APSDecReqA : Subsystem
  APSOpenPTG : Subsystem
  APSReq : Subsystem
  APSStaSystem : Subsystem
  Byte_0 : Subsystem
  Byte_1 : Subsystem
  Byte_{8..15} (8 alike) : Constant  Value=ZERO_INT
  Byte_2 : Subsystem
  Byte_3 : Subsystem
  Byte_4 : Subsystem
  Byte_5 : Subsystem
  Byte_6 : Subsystem
  Byte_7 : Subsystem
  CAASSta : Subsystem
  CRC8_IfAction_Tx : Subsystem  AncestorBlock=FVT_lib/hal/CRC8_IfAction_Tx
      mask help: MeasumentTrigerEvent
      mask Display: fprintf('CRC8_IfAction');
  Constant : Constant  Value=KHAL_CAN6FD6APS3E2E_flg
  Constant1 : Constant  Value=0xE5
  Constant2 : Constant  Value=0x86
  Constant3 : Constant  Value=KHAL_CAN6FD6APS3E2E_flg
  Constant4 : Constant  Value=KHAL_CAN6FD6APS3E2E_flg
  FDCVMCAPSAngleTarget : Subsystem
  FDCVMCAPSRqEPSCtrl : Subsystem
  FDCVMCAPSVRqEPSCtrl : Subsystem
  Ground : Ground
  Ground1 : Ground
  Ground2 : Ground
  Mux2 : Mux  Inputs=15
  RollingCounter_IfAction : FVT_lib/hal/RollingCounter_IfAction
  RollingCounter_IfAction1 : FVT_lib/hal/RollingCounter_IfAction
  SPTGDet : Subsystem
  SPTGSta : Subsystem
  Terminator : Terminator
  bus_creator : BusCreator  Inputs=13  OutDataTypeStr=Bus: DT_CAN6_SG_FD6_APS3  NonVirtualBus=on
  bus_selector : BusSelector  OutputSignals=VOUTP_APSOpenPTG_flg
  bus_selector1 : BusSelector  OutputSignals=VOUTP_APSDecReqA_flg
  bus_selector10 : BusSelector  OutputSignals=VOUTP_FDCVMCAPSRqEPSCtrl_flg
  bus_selector11 : BusSelector  OutputSignals=VOUTP_APSOpenPTG_flg
  bus_selector12 : BusSelector  OutputSignals=VOUTP_APSDecReq_mps2
  bus_selector13 : BusSelector  OutputSignals=VOUTP_APSDecReqA_flg
  bus_selector14 : BusSelector  OutputSignals=VOUTP_APSReq_enum
  bus_selector15 : BusSelector  OutputSignals=VOUTP_APSStaSys_enum
  bus_selector16 : BusSelector  OutputSignals=VOUTP_CAASSta_enum
  bus_selector17 : BusSelector  OutputSignals=VOUTP_FDCVMCAPSAngleTarget_deg
  bus_selector18 : BusSelector  OutputSignals=VOUTP_FDCVMCAPSRqEPSCtrl_flg
  bus_selector19 : BusSelector  OutputSignals=VOUTP_FDCVMCAPSVRqEPSCtrl_flg
  bus_selector2 : BusSelector  OutputSignals=VOUTP_APSReq_enum
  bus_selector20 : BusSelector  OutputSignals=VOUTP_SPTGDet_flg
  bus_selector3 : BusSelector  OutputSignals=VOUTP_CAASSta_enum
  bus_selector4 : BusSelector  OutputSignals=VOUTP_APSDecReq_mps2
  bus_selector5 : BusSelector  OutputSignals=VOUTP_FDCVMCAPSAngleTarget_deg
  bus_selector6 : BusSelector  OutputSignals=VOUTP_FDCVMCAPSAngleTarget_deg
  bus_selector7 : BusSelector  OutputSignals=VOUTP_APSStaSys_enum
  bus_selector8 : BusSelector  OutputSignals=VOUTP_FDCVMCAPSVRqEPSCtrl_flg
  bus_selector9 : BusSelector  OutputSignals=VOUTP_SPTGDet_flg
  FD6_APS3 : Outport
  wires:
  BSCP_outputs/1 -> [BSCP_outputs]
  BOUTP_outputs/1 -> [BOUTP_outputs]
  [CAN6_APS3_LifeCount] -> bus_creator/1  "CAN6_APS3_LifeCount"
  [CAN6_APS3_checksum] -> bus_creator/2  "CAN6_APS3_checksum"
  [CAN6_APSOpenPTG] -> bus_creator/3  "CAN6_APSOpenPTG"
  [CAN6_APS_DecReq] -> bus_creator/4  "CAN6_APS_DecReq"
  [CAN6_APS_DecReq_A] -> bus_creator/5  "CAN6_APS_DecReq_A"
  [CAN6_APS_Req] -> bus_creator/6  "CAN6_APS_Req"
  [CAN6_APS_Sta_System] -> bus_creator/7  "CAN6_APS_Sta_System"
  [CAN6_CAAS_Sta] -> bus_creator/8  "CAN6_CAAS_Sta"
  [CAN6_FDC_VMC_APS_Angle_Target] -> bus_creator/9  "CAN6_FDC_VMC_APS_Angle_Target"
  [CAN6_FDC_VMC_APS_Rq_EPS_Ctrl] -> bus_creator/10  "CAN6_FDC_VMC_APS_Rq_EPS_Ctrl"
  [CAN6_FDC_VMC_APS_V_Rq_EPS_Ctrl] -> bus_creator/11  "CAN6_FDC_VMC_APS_V_Rq_EPS_Ctrl"
  [CAN6_SPTGDet] -> bus_creator/12  "CAN6_SPTGDet"
  [CAN6_SPTG_Sta] -> bus_creator/13  "CAN6_SPTG_Sta"
  bus_creator/1 -> FD6_APS3/1
  APS3LifeCount/1(CAN6_APS3_LifeCount) -> [CAN6_APS3_LifeCount]
  APS3checksum/1(CAN6_APS3_checksum) -> [CAN6_APS3_checksum]
  APSOpenPTG/1(CAN6_APSOpenPTG) -> [CAN6_APSOpenPTG]
  APSDecReq/1(CAN6_APS_DecReq) -> [CAN6_APS_DecReq]
  APSDecReqA/1(CAN6_APS_DecReq_A) -> [CAN6_APS_DecReq_A]
  APSReq/1(CAN6_APS_Req) -> [CAN6_APS_Req]
  APSStaSystem/1(CAN6_APS_Sta_System) -> [CAN6_APS_Sta_System]
  CAASSta/1(CAN6_CAAS_Sta) -> [CAN6_CAAS_Sta]
  FDCVMCAPSAngleTarget/1(CAN6_FDC_VMC_APS_Angle_Target) -> [CAN6_FDC_VMC_APS_Angle_Target]
  FDCVMCAPSRqEPSCtrl/1(CAN6_FDC_VMC_APS_Rq_EPS_Ctrl) -> [CAN6_FDC_VMC_APS_Rq_EPS_Ctrl]
  FDCVMCAPSVRqEPSCtrl/1(CAN6_FDC_VMC_APS_V_Rq_EPS_Ctrl) -> [CAN6_FDC_VMC_APS_V_Rq_EPS_Ctrl]
  SPTGDet/1(CAN6_SPTGDet) -> [CAN6_SPTGDet]
  SPTGSta/1(CAN6_SPTG_Sta) -> [CAN6_SPTG_Sta]
  Byte_0/1(Byte_0) -> Terminator/1
  Byte_1/1(Byte_1) -> [Byte_1]
  Byte_2/1(Byte_2) -> [Byte_2]
  Byte_3/1(Byte_3) -> [Byte_3]
  Byte_4/1(Byte_4) -> [Byte_4]
  Byte_5/1(Byte_5) -> [Byte_5]
  Byte_6/1(Byte_6) -> [Byte_6]
  Byte_7/1(Byte_7) -> [Byte_7]
  Byte_8/1 -> [Byte_8]
  Byte_9/1 -> [Byte_9]
  Byte_10/1 -> [Byte_10]
  Byte_11/1 -> [Byte_11]
  Byte_12/1 -> [Byte_12]
  Byte_13/1 -> [Byte_13]
  Byte_14/1 -> [Byte_14]
  Byte_15/1 -> [Byte_15]
  Mux2/1 -> CRC8_IfAction_Tx/4(RawData)
  Constant/1 -> CRC8_IfAction_Tx/1(CAN_E2E_flg)
  Constant1/1 -> CRC8_IfAction_Tx/2(DataID1)
  Constant2/1 -> CRC8_IfAction_Tx/3(DataID2)
  CRC8_IfAction_Tx/1(CRC8) -> [APS3_checksum]
  Ground/1 -> Byte_0/1(APS3_checksum)
  [Byte_1] -> Mux2/1
  RollingCounter_IfAction/1 -> Byte_1/1(APS3_LifeCount)
  Constant3/1 -> RollingCounter_IfAction/1
  [Byte_2] -> Mux2/2
  bus_selector/1 -> Byte_2/1(APSOpenPTG)  "<VOUTP_APSOpenPTG_flg>"
  [BOUTP_outputs] -> bus_selector/1
  bus_selector1/1 -> Byte_2/2(APS_DecReq_A)  "<VOUTP_APSDecReqA_flg>"
  [BOUTP_outputs] -> bus_selector1/1
  bus_selector2/1 -> Byte_2/3(APS_Req)  "<VOUTP_APSReq_enum>"
  [BOUTP_outputs] -> bus_selector2/1
  bus_selector3/1 -> Byte_2/4(CAAS_Sta)  "<VOUTP_CAASSta_enum>"
  [BOUTP_outputs] -> bus_selector3/1
  [Byte_3] -> Mux2/3
  bus_selector4/1 -> Byte_3/1(APS_DecReq)  "<VOUTP_APSDecReq_mps2>"
  [BOUTP_outputs] -> bus_selector4/1
  [Byte_4] -> Mux2/4
  bus_selector5/1 -> Byte_4/1(FDC_VMC_APS_Angle_Target)  "<VOUTP_FDCVMCAPSAngleTarget_deg>"
  [BOUTP_outputs] -> bus_selector5/1
  [Byte_5] -> Mux2/5
  bus_selector6/1 -> Byte_5/1(FDC_VMC_APS_Angle_Target)  "<VOUTP_FDCVMCAPSAngleTarget_deg>"
  [BOUTP_outputs] -> bus_selector6/1
  [Byte_6] -> Mux2/6
  bus_selector7/1 -> Byte_6/1(APS_Sta_System)  "<VOUTP_APSStaSys_enum>"
  [BOUTP_outputs] -> bus_selector7/1
  bus_selector8/1 -> Byte_6/2(FDC_VMC_APS_V_Rq_EPS_Ctrl)  "<VOUTP_FDCVMCAPSVRqEPSCtrl_flg>"
  [BOUTP_outputs] -> bus_selector8/1
  bus_selector9/1 -> Byte_6/3(SPTGDet)  "<VOUTP_SPTGDet_flg>"
  [BOUTP_outputs] -> bus_selector9/1
  Ground1/1 -> Byte_6/4(SPTG_Sta)
  [Byte_7] -> Mux2/7
  bus_selector10/1 -> Byte_7/1(FDC_VMC_APS_Rq_EPS_Ctrl)  "<VOUTP_FDCVMCAPSRqEPSCtrl_flg>"
  [BOUTP_outputs] -> bus_selector10/1
  [Byte_8] -> Mux2/8
  [Byte_9] -> Mux2/9
  [Byte_10] -> Mux2/10
  [Byte_11] -> Mux2/11
  [Byte_12] -> Mux2/12
  [Byte_13] -> Mux2/13
  [Byte_14] -> Mux2/14
  [Byte_15] -> Mux2/15
  RollingCounter_IfAction1/1 -> APS3LifeCount/1(APS3LifeCount)
  Constant4/1 -> RollingCounter_IfAction1/1
  [APS3_checksum] -> APS3checksum/1(APS3checksum)
  bus_selector11/1 -> APSOpenPTG/1(APSOpenPTG)  "<VOUTP_APSOpenPTG_flg>"
  [BOUTP_outputs] -> bus_selector11/1
  bus_selector12/1 -> APSDecReq/1(APSDecReq)  "<VOUTP_APSDecReq_mps2>"
  [BOUTP_outputs] -> bus_selector12/1
  bus_selector13/1 -> APSDecReqA/1(APSDecReqA)  "<VOUTP_APSDecReqA_flg>"
  [BOUTP_outputs] -> bus_selector13/1
  bus_selector14/1 -> APSReq/1(APSReq)  "<VOUTP_APSReq_enum>"
  [BOUTP_outputs] -> bus_selector14/1
  bus_selector15/1 -> APSStaSystem/1(APSStaSystem)  "<VOUTP_APSStaSys_enum>"
  [BOUTP_outputs] -> bus_selector15/1
  bus_selector16/1 -> CAASSta/1(CAASSta)  "<VOUTP_CAASSta_enum>"
  [BOUTP_outputs] -> bus_selector16/1
  bus_selector17/1 -> FDCVMCAPSAngleTarget/1(FDCVMCAPSAngleTarget)  "<VOUTP_FDCVMCAPSAngleTarget_deg>"
  [BOUTP_outputs] -> bus_selector17/1
  bus_selector18/1 -> FDCVMCAPSRqEPSCtrl/1(FDCVMCAPSRqEPSCtrl)  "<VOUTP_FDCVMCAPSRqEPSCtrl_flg>"
  [BOUTP_outputs] -> bus_selector18/1
  bus_selector19/1 -> FDCVMCAPSVRqEPSCtrl/1(FDCVMCAPSVRqEPSCtrl)  "<VOUTP_FDCVMCAPSVRqEPSCtrl_flg>"
  [BOUTP_outputs] -> bus_selector19/1
  bus_selector20/1 -> SPTGDet/1(SPTGDet)  "<VOUTP_SPTGDet_flg>"
  [BOUTP_outputs] -> bus_selector20/1
  Ground2/1 -> SPTGSta/1(SPTGSta)

== system halout/HAL_OUT/CAN6/FD6_APS3_Tx ==
  TxReq : Inport
  Chart : Stateflow chart  TreatAsAtomicUnit=on
  Constant : Constant  Value=C_TASK_5MS_S
  Constant3 : Constant  Value=CycleTime
  Data Type Conversion : DataTypeConversion  OutDataTypeStr=uint16
  Divide : Product  Inputs=*/
  Gain : Gain  Gain=0.001
  TxTrigger : Outport
  wires:
  Data Type Conversion/1 -> Chart/2(CycleCnt)
  Constant3/1 -> Gain/1
  Gain/1 -> Divide/1
  Chart/1(TxTrigger()) -> TxTrigger/1
  Divide/1 -> Data Type Conversion/1
  TxReq/1 -> Chart/1(TxReq)
  Constant/1 -> Divide/2
